simulink model "Simul3_contr2"  (R2023a)
settings: Solver=VariableStepAuto  StartTime=0.0  StopTime=10.0  RelTol=1e-3
values from neighbouring files (symbols this model uses):
  A = [[-3.333 0 -1.3333];[2 -2 0];[0 4.7727 -0.04545]]    [Controlador_t3.m]    (also in lab2_controle2.m = [[0 1 0];[981.0001 0 -2.8814];[0 0 -100]]; trab3_controle2.m; trabalho1_controle2.m = [[0 1];[0 0]])
  b1 = [3.3333;0;0]    [Controlador_t3.m]    (also in trab3_controle2.m)
  c = [0 0 1]    [Controlador_t3.m]    (also in lab2_controle2.m = [1 0 0]; trab3_controle2.m; trabalho1_controle2.m = [1,0])
undefined symbols (not defined in the file or in its folder): K
settings Model: Creator=wesle  LastModifiedBy=wesle

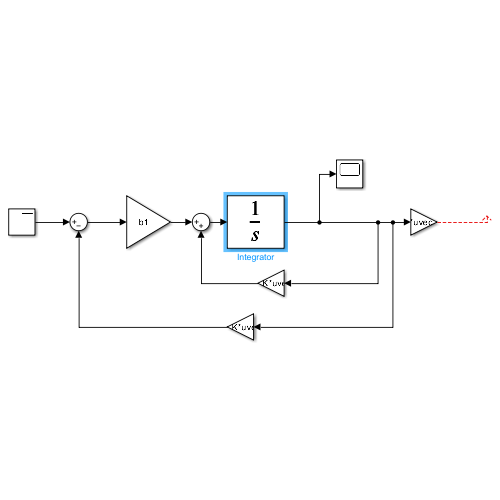
[thumbnail: Simulink's stored preview of the top-level diagram]
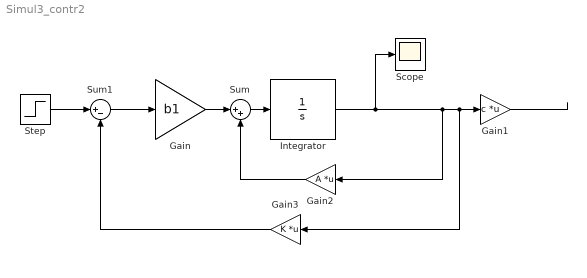
== system Simul3_contr2 ==
  Gain : Gain  Gain=b1
  Gain1 : Gain  Gain=c  Multiplication=Matrix(K*u) (u vector)
  Gain2 : Gain  Gain=A  Multiplication=Matrix(K*u) (u vector)
  Gain3 : Gain  Gain=K  Multiplication=Matrix(K*u) (u vector)
  Integrator : Integrator  InitialCondition=[0;0;0]
  Scope : Scope
  Step : Step  SampleTime=0
  Sum : Sum  Inputs=|++
  Sum1 : Sum  Inputs=|+-
  wires:
  Gain1/1 -> ?
  Integrator/1 -> Scope/1, Gain3/1, Gain1/1, Gain2/1
  Gain/1 -> Sum/1
  Sum/1 -> Integrator/1
  Gain2/1 -> Sum/2
  Step/1 -> Sum1/1
  Sum1/1 -> Gain/1
  Gain3/1 -> Sum1/2
